simulink model "Model2"  (R2018b)
settings: Solver=ode4  StartTime=0.0  StopTime=tend  FixedStep=dt  RelTol=1e-3
values from neighbouring files (symbols this model uses):
  Bm = 8.6457e-06    [CompareMeasurementModel.m]    (also in ForcedResponse.m; StateSpaceFix.m; SystemEstimateFullN.m; SystemEstimateGammaN.m = 0.0040665)
  Dc = 9.4912e-6    (= 9.4912e-06)    [CompareMeasurementModel.m]    (also in ForcedResponse.m = 8.0176e-06; StateSpaceFix.m = 8.0176e-06; SystemEstimateFullN.m = 0)
  F = 1.3447e-07    [CompareMeasurementModel.m]    (also in ForcedResponse.m; StateSpaceFix.m; SystemEstimateFullN.m; SystemEstimateGammaN.m = 6.3647e-07)
  Freq = 2    [ForcedResponse.m]    (also in StateSpaceFix.m = 1)
  gamma = 1.4811e-09    [CompareMeasurementModel.m]    (also in ForcedResponse.m; StateSpaceFix.m; SystemEstimateFullN.m; SystemEstimateGammaN.m = 8.9133e-10)
  I = 0.012124    [CompareMeasurementModel.m]    (also in ForcedResponse.m = 0.00046323; StateSpaceFix.m = 0.00046323; SystemEstimateFullN.m = 0)
  init = [0 ;0 ;0]    [CompareMeasurementModel.m]    (also in ForcedResponse.m; StateSpaceFix.m; SystemEstimateFullN.m; SystemEstimateGammaN.m = [Pplot(1,1)/(Rg*T/V0) ;0 ;0])
  Jm = 3.0991e-09    [CompareMeasurementModel.m]    (also in ForcedResponse.m; StateSpaceFix.m; SystemEstimateFullN.m; SystemEstimateGammaN.m = 0.00030736)
  L = 0.509    [CompareMeasurementModel.m]    (also in ForcedResponse.m; StateSpaceFix.m; SystemEstimateFullN.m; SystemEstimateGammaN.m)
  N = 73.6905    [CompareMeasurementModel.m]    (also in ForcedResponse.m = 8.8595; StateSpaceFix.m = 8.8595; SystemEstimateFullN.m = 1)
  P = 0.0011648    [CompareMeasurementModel.m]    (also in ForcedResponse.m = 0.00015249; StateSpaceFix.m = 0.00015249; SystemEstimateFullN.m = 1)
  Pend = 1000    [CompareMeasurementModel.m]    (also in ForcedResponse.m = 20000; StateSpaceFix.m = 30000; SystemEstimateFullN.m = 100)
  Period = Tpc*SampleRate*2    (= 20)    [CompareMeasurementModel.m]    (also in ForcedResponse.m = 25; StateSpaceFix.m = 25; SystemEstimateFullN.m; SystemEstimateGammaN.m)
  RatedRatio = 0.0049254    [CompareMeasurementModel.m]    (also in ForcedResponse.m; StateSpaceFix.m; SystemEstimateFullN.m)
  Res = 10    [CompareMeasurementModel.m]    (also in ForcedResponse.m; StateSpaceFix.m; SystemEstimateFullN.m; SystemEstimateGammaN.m)
  Rg = 287.058    [CompareMeasurementModel.m]    (also in ForcedResponse.m; StateSpaceFix.m; SystemEstimateFullN.m; SystemEstimateGammaN.m)
  T = 293.15    [CompareMeasurementModel.m]    (also in ForcedResponse.m; StateSpaceFix.m; SystemEstimateFullN.m; SystemEstimateGammaN.m)
  tau0 = RatedRatio    (= 0.0049254)    [CompareMeasurementModel.m]    (also in ForcedResponse.m; StateSpaceFix.m; SystemEstimateFullN.m; SystemEstimateGammaN.m = 0.53226)
  tstart = Tplot(k-Start+1,1)    [CompareMeasurementModel.m]    (also in ForcedResponse.m = 1; StateSpaceFix.m = 1; SystemEstimateFullN.m; SystemEstimateGammaN.m = 0)
  V0 = 7.658796956e-5    (= 7.658796956e-05)    [CompareMeasurementModel.m]    (also in ForcedResponse.m; StateSpaceFix.m; SystemEstimateFullN.m; SystemEstimateGammaN.m)
  Vboundlower = 0    [ForcedResponse.m]    (also in StateSpaceFix.m)
  Vboundupper = 5    [ForcedResponse.m]    (also in StateSpaceFix.m)
  Vend = V    [CompareMeasurementModel.m]    (also in ForcedResponse.m = 1.5; StateSpaceFix.m = 1.5; SystemEstimateFullN.m; SystemEstimateGammaN.m = 0)
  Vr = 1    [CompareMeasurementModel.m]    (also in ForcedResponse.m; StateSpaceFix.m; SystemEstimateFullN.m; SystemEstimateGammaN.m = 5.48)
  Vs = 1.3    [ForcedResponse.m]    (also in StateSpaceFix.m; SystemEstimateGammaN.m)
  Z = 1.553807*10^(-6)    (= 1.553807e-06)    [CompareMeasurementModel.m]    (also in ForcedResponse.m; StateSpaceFix.m; SystemEstimateFullN.m; SystemEstimateGammaN.m)
libraries: simulink x7
settings Model: Creator=s152155  LastModifiedBy=s152155

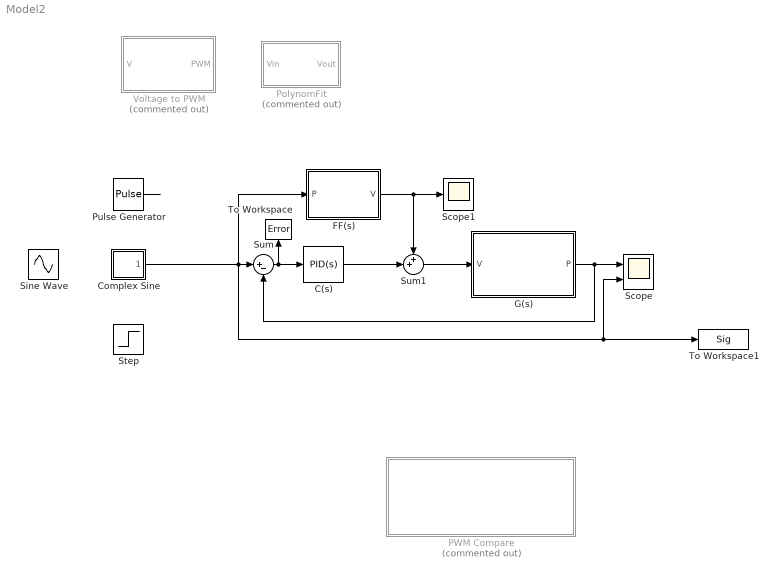
== system Model2 ==
  C(s) : simulink/Continuous/PID Controller  Controller=PID  Form=Parallel  TimeDomain=Continuous-time  SampleTime=-1  IntegratorMethod=Forward Euler  FilterMethod=Forward Euler  ControllerParametersSource=internal  P=P  I=I  D=Dc  UseFilter=on  N=N  TunerSelectOption=Transfer Function Based (PID Tuner App)  InitialConditionSource=internal  InitialConditionForIntegrator=0  InitialConditionForFilter=0  DifferentiatorICPrevScaledInput=0  ExternalReset=none  TrackingMode=off  Kt=1  LimitOutput=off  UpperSaturationLimit=inf  LowerSaturationLimit=-inf  LinearizeAsGain=on  AntiWindupMode=none  Kb=1  POutMin=[]  POutMax=[]  IOutMin=[]  IOutMax=[]  DOutMin=[]  DOutMax=[]  NOutMin=[0]  NOutMax=[0]  SumOutMin=[]  SumOutMax=[]  SaturationOutMin=[]  SaturationOutMax=[]  PParamMin=[]  PParamMax=[]  IParamMin=[]  IParamMax=[]  DParamMin=[]  DParamMax=[]  NParamMin=[]  NParamMax=[]  KbParamMin=[]  KbParamMax=[]  KtParamMin=[]  KtParamMax=[]  KbOutMin=[]  KbOutMax=[]  KtOutMin=[]  KtOutMax=[]  IntegratorOutMin=[]  IntegratorOutMax=[]  FilterOutMin=[]  FilterOutMax=[]  SumI1OutMin=[]  SumI1OutMax=[]  SumI2OutMin=[]  SumI2OutMax=[]  SumI3OutMin=[]  SumI3OutMax=[]  SumI4OutMin=[]  SumI4OutMax=[]  SumDOutMin=[]  SumDOutMax=[]  DifferentiatorOutMin=[]  DifferentiatorOutMax=[]  FilterDiffOutCoefMin=[]  FilterDiffOutCoefMax=[]  ReciprocalOutMin=[]  ReciprocalOutMax=[]  SumDenOutMin=[]  SumDenOutMax=[]  SumNumOutMin=[]  SumNumOutMax=[]  DivideOutMin=[]  DivideOutMax=[]  IntegratorContinuousStateAttributes=''  IntegratorStateMustResolveToSignalObject=off  IntegratorRTWStateStorageClass=Auto  FilterContinuousStateAttributes=''  FilterStateMustResolveToSignalObject=off  FilterRTWStateStorageClass=Auto  ParallelPVariant=InternalParameters  IdealPVariant=Disabled  IVariant=InternalParameters  DVariant=InternalParameters  IntegratorVariant=Continuous  SatVariant=Disabled  AWVariant=Passthrough  PCopyVariant=Disabled  TRVariant=Disabled  FdbkBlocksVariant=Forward  IdealPFdbkVariant=Disabled  SatFdbkVariant=Disabled  DerivativeFilterVariant=ContFilter  NVariant=InternalParameters  NCopyVariant=Disabled  FilterICVariant=InternalICsFilter  IntegratorICVariant=InternalICs  ExternalResetVariant=Disabled  TRSumVariant=Passthrough  SumFdbkVariant=Disabled  SumVariant=Sum_PID
  "Complex Sine " : Subsystem
  FF(s) : Subsystem
  G(s) : Subsystem
  PWM Compare : Subsystem  Commented=on
  "PolynomFit " : Subsystem  Commented=on
  Pulse Generator : DiscretePulseGenerator  PulseType=Time based  Amplitude=Vend  Period=Period  PulseWidth=50  PhaseDelay=tstart
  Scope : Scope  NumInputPorts=2
  Scope1 : Scope
  Sine Wave : Sin  Amplitude=Pend/2  Bias=Pend/2  Frequency=Freq  SampleTime=0
  Step : Step  Time=tstart  After=Pend  SampleTime=0
  Sum : Sum  Inputs=|+-
  Sum1 : Sum  Inputs=++|
  To Workspace : ToWorkspace  VariableName=Error  SaveFormat=Timeseries  SampleTime=-1
  To Workspace1 : ToWorkspace  VariableName=Sig  SaveFormat=Timeseries  SampleTime=-1
  Voltage to PWM : Subsystem  Commented=on
  wires:
  G(s)/1(P) -> Scope/1, Sum/2
  "Complex Sine "/1(Pref) -> To Workspace1/1, Scope/2, FF(s)/1(P), Sum/1
  Sum/1 -> C(s)/1, To Workspace/1
  C(s)/1 -> Sum1/2
  Pulse Generator/1 -> ?
  FF(s)/1(V) -> Sum1/1, Scope1/1
  Sum1/1 -> G(s)/1(V)

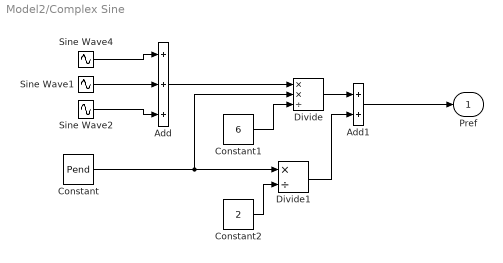
== system Model2/Complex Sine  ==
  Add : Sum  Inputs=3
  Add1 : Sum
  Constant : Constant  Value=Pend
  Constant1 : Constant  Value=6
  Constant2 : Constant  Value=2
  Divide : Product  Inputs=**/
  Divide1 : Product  Inputs=*/
  Sine Wave1 : Sin  Frequency=2*Freq  SampleTime=0
  Sine Wave2 : Sin  Frequency=3*Freq  SampleTime=0
  Sine Wave4 : Sin  Frequency=Freq  SampleTime=0
  Pref : Outport
  wires:
  Divide1/1 -> Add1/2
  Constant/1 -> Divide/2, Divide1/1
  Sine Wave2/1 -> Add/3
  Constant1/1 -> Divide/3
  Sine Wave4/1 -> Add/1
  Sine Wave1/1 -> Add/2
  Divide/1 -> Add1/1
  Constant2/1 -> Divide1/2
  Add/1 -> Divide/1
  Add1/1 -> Pref/1

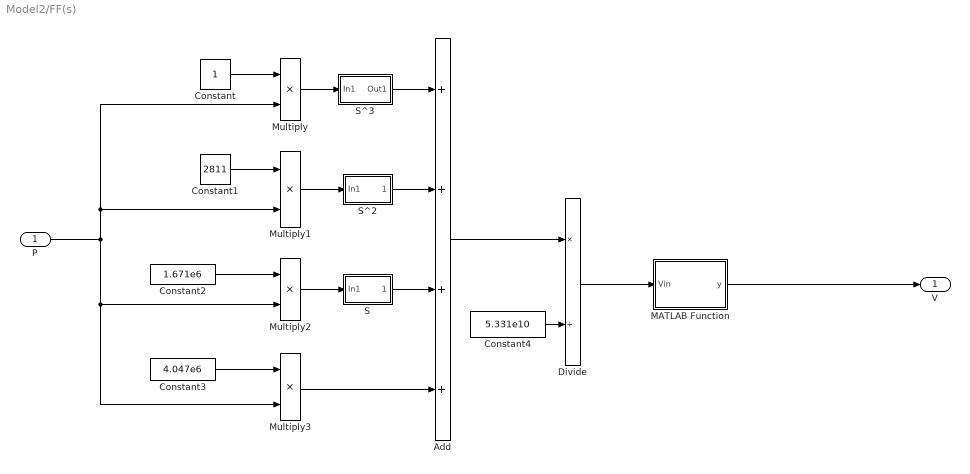
== system Model2/FF(s) ==
  P : Inport
  Add : Sum  Inputs=4
  Constant : Constant
  Constant1 : Constant  Value=2811
  Constant2 : Constant  Value=1.671e6
  Constant3 : Constant  Value=4.047e6
  Constant4 : Constant  Value=5.331e10
  Divide : Product  Inputs=*/
  MATLAB Function : MATLAB Function  TreatAsAtomicUnit=on
  Multiply{,1..3} (4 alike) : Product
  S : Subsystem
  S^2 : Subsystem
  S^3 : Subsystem
  V : Outport
  wires:
  S^3/1(Out1) -> Add/1
  S^2/1(Out1) -> Add/2
  S/1(Out1) -> Add/3
  Constant3/1 -> Multiply3/1
  Constant2/1 -> Multiply2/1
  Constant1/1 -> Multiply1/1
  Constant/1 -> Multiply/1
  Constant4/1 -> Divide/2
  Add/1 -> Divide/1
  P/1 -> Multiply3/2, Multiply2/2, Multiply1/2, Multiply/2
  Multiply/1 -> S^3/1(In1)
  Multiply1/1 -> S^2/1(In1)
  Multiply2/1 -> S/1(In1)
  Multiply3/1 -> Add/4
  Divide/1 -> MATLAB Function/1(Vin)
  MATLAB Function/1(y) -> V/1

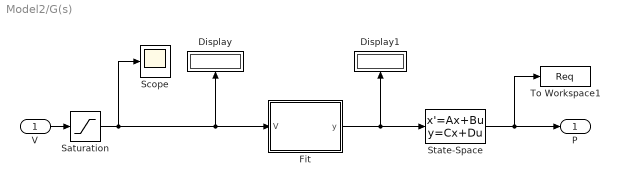
== system Model2/G(s) ==
  V : Inport
  Display : Display
  Display1 : Display
  Fit : MATLAB Function  TreatAsAtomicUnit=on
  Saturation : Saturate  UpperLimit=Vboundupper  LowerLimit=Vboundlower
  Scope : Scope
  State-Space : StateSpace  A=[-gamma*Rg*T/V0 0 Z; 0 -Res/L -Res*RatedRatio/(L); -(F/Jm)*(Rg*T/V0) Res*RatedRatio/(Jm) -Bm/Jm]  B=[0; 1/L; 0]  C=[Rg*T/V0 0 0]  D=0  InitialCondition=init  ContinuousStateAttributes="{'mass',  'current', 'rotationalvelocity'}"
  To Workspace1 : ToWorkspace  VariableName=Req  SaveFormat=Timeseries  SampleTime=-1
  P : Outport
  wires:
  State-Space/1 -> To Workspace1/1, P/1
  V/1 -> Saturation/1
  Saturation/1 -> Scope/1, Display/1, Fit/1(V)
  Fit/1(y) -> Display1/1, State-Space/1

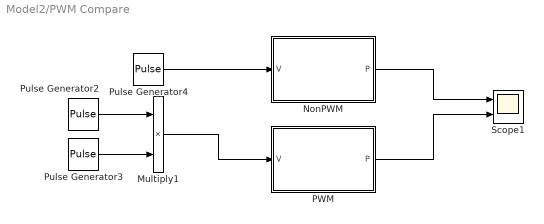
== system Model2/PWM Compare ==
  " NonPWM" : Subsystem
  Multiply1 : Product
  PWM : Subsystem
  Pulse Generator2 : DiscretePulseGenerator  PulseType=Time based  Amplitude=5  Period=25  PulseWidth=50
  Pulse Generator3 : DiscretePulseGenerator  PulseType=Time based  Period=0.01  PulseWidth=60
  Pulse Generator4 : DiscretePulseGenerator  PulseType=Time based  Amplitude=3  Period=Period  PulseWidth=50
  Scope1 : Scope  NumInputPorts=2
  wires:
  Multiply1/1 -> PWM/1(V)
  Pulse Generator3/1 -> Multiply1/2
  Pulse Generator2/1 -> Multiply1/1
  PWM/1(P) -> Scope1/2
  " NonPWM"/1(P) -> Scope1/1
  Pulse Generator4/1 -> " NonPWM"/1(V)

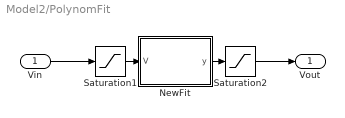
== system Model2/PolynomFit  ==
  Vin : Inport
  "NewFit " : MATLAB Function  TreatAsAtomicUnit=on
  Saturation1 : Saturate  UpperLimit=5  LowerLimit=1.35
  Saturation2 : Saturate  UpperLimit=inf  LowerLimit=0
  Vout : Outport
  wires:
  Saturation1/1 -> "NewFit "/1(V)
  "NewFit "/1(y) -> Saturation2/1
  Vin/1 -> Saturation1/1
  Saturation2/1 -> Vout/1

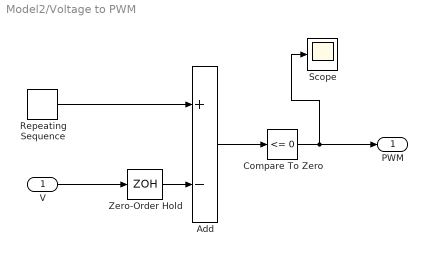
== system Model2/Voltage to PWM ==
  V : Inport
  Add : Sum  Inputs=+-
  Compare To Zero : simulink/Logic and Bit Operations/Compare To Zero  relop=<=  OutDataTypeStr=boolean
  Repeating Sequence : simulink/Sources/Repeating Sequence  rep_seq_t=[0 1]  rep_seq_y=[0 1]
  Scope : Scope
  Zero-Order Hold : ZeroOrderHold  SampleTime=-1
  PWM : Outport
  wires:
  V/1 -> Zero-Order Hold/1
  Zero-Order Hold/1 -> Add/2
  Add/1 -> Compare To Zero/1
  Compare To Zero/1 -> Scope/1, PWM/1
  Repeating Sequence/1 -> Add/1

== system Model2/FF(s)/S ==
  In1 : Inport
  Derivative5 : Derivative
  Out1 : Outport
  wires:
  Derivative5/1 -> Out1/1
  In1/1 -> Derivative5/1

== system Model2/FF(s)/S^2 ==
  In1 : Inport
  Derivative3 : Derivative
  Derivative4 : Derivative
  Out1 : Outport
  wires:
  Derivative4/1 -> Out1/1
  Derivative3/1 -> Derivative4/1
  In1/1 -> Derivative3/1

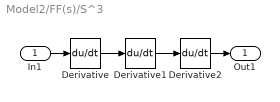
== system Model2/FF(s)/S^3 ==
  In1 : Inport
  Derivative : Derivative
  Derivative1 : Derivative
  Derivative2 : Derivative
  Out1 : Outport
  wires:
  Derivative2/1 -> Out1/1
  Derivative1/1 -> Derivative2/1
  In1/1 -> Derivative/1
  Derivative/1 -> Derivative1/1

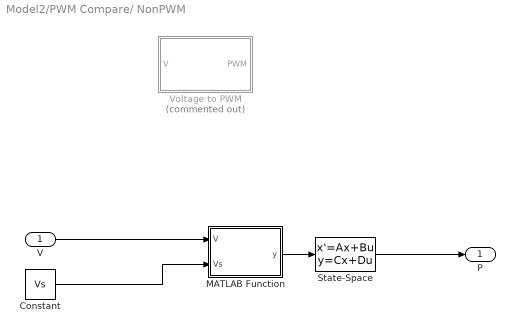
== system Model2/PWM Compare/ NonPWM ==
  V : Inport
  Constant : Constant  Value=Vs
  MATLAB Function : MATLAB Function  TreatAsAtomicUnit=on
  State-Space : StateSpace  A=[-gamma*Rg*T/V0 0 Z; 0 -Res/L -Res*tau0/(L*Vr); -(F/Jm)*(Rg*T/V0) Res*tau0/(Jm*Vr) -Bm/Jm]  B=[0; 1/L; 0]  C=[Rg*T/V0 0 0]  D=0  InitialCondition=init  ContinuousStateAttributes="{'mass',  'current', 'rotationalvelocity'}"
  Voltage to PWM : Subsystem  Commented=on
  P : Outport
  wires:
  State-Space/1 -> P/1
  MATLAB Function/1(y) -> State-Space/1
  V/1 -> MATLAB Function/1(V)
  Constant/1 -> MATLAB Function/2(Vs)

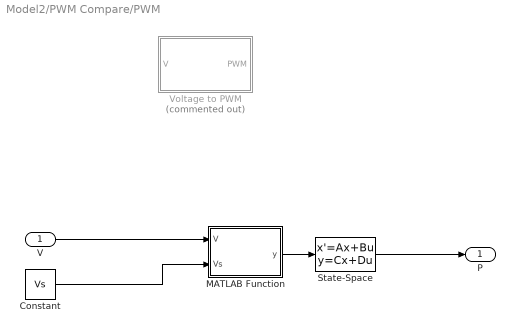
== system Model2/PWM Compare/PWM ==
  V : Inport
  Constant : Constant  Value=Vs
  MATLAB Function : MATLAB Function  TreatAsAtomicUnit=on
  State-Space : StateSpace  A=[-gamma*Rg*T/V0 0 Z; 0 -Res/L -Res*tau0/(L*Vr); -(F/Jm)*(Rg*T/V0) Res*tau0/(Jm*Vr) -Bm/Jm]  B=[0; 1/L; 0]  C=[Rg*T/V0 0 0]  D=0  InitialCondition=init  ContinuousStateAttributes="{'mass',  'current', 'rotationalvelocity'}"
  Voltage to PWM : Subsystem  Commented=on
  P : Outport
  wires:
  State-Space/1 -> P/1
  MATLAB Function/1(y) -> State-Space/1
  V/1 -> MATLAB Function/1(V)
  Constant/1 -> MATLAB Function/2(Vs)

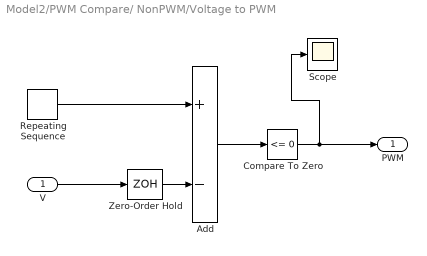
== system Model2/PWM Compare/ NonPWM/Voltage to PWM ==
  V : Inport
  Add : Sum  Inputs=+-
  Compare To Zero : simulink/Logic and Bit Operations/Compare To Zero  relop=<=  OutDataTypeStr=boolean
  Repeating Sequence : simulink/Sources/Repeating Sequence  rep_seq_t=[0 1]  rep_seq_y=[0 1]
  Scope : Scope
  Zero-Order Hold : ZeroOrderHold  SampleTime=-1
  PWM : Outport
  wires:
  V/1 -> Zero-Order Hold/1
  Zero-Order Hold/1 -> Add/2
  Add/1 -> Compare To Zero/1
  Compare To Zero/1 -> Scope/1, PWM/1
  Repeating Sequence/1 -> Add/1

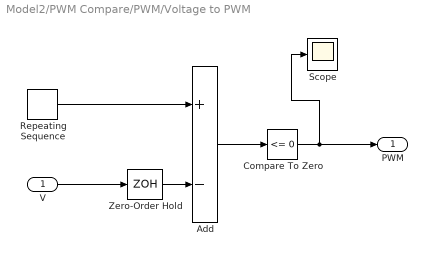
== system Model2/PWM Compare/PWM/Voltage to PWM ==
  V : Inport
  Add : Sum  Inputs=+-
  Compare To Zero : simulink/Logic and Bit Operations/Compare To Zero  relop=<=  OutDataTypeStr=boolean
  Repeating Sequence : simulink/Sources/Repeating Sequence  rep_seq_t=[0 1]  rep_seq_y=[0 1]
  Scope : Scope
  Zero-Order Hold : ZeroOrderHold  SampleTime=-1
  PWM : Outport
  wires:
  V/1 -> Zero-Order Hold/1
  Zero-Order Hold/1 -> Add/2
  Add/1 -> Compare To Zero/1
  Compare To Zero/1 -> Scope/1, PWM/1
  Repeating Sequence/1 -> Add/1

== matlab function Model2/PWM Compare/ NonPWM/MATLAB Function ==
  data: V input; y output; Vs input
function y = Vmin(V, Vs)
if V >= Vs
elseif V<Vs
    V = 0;
elseif V<-Vs
    V = -V;
end
y = V;

== matlab function Model2/G(s)/Fit ==
  data: V input; y output
function y = Vmin(V)
z = 15000;
if V >= 1.1
elseif V<1.1
    V = 0;
elseif V<-1.1
    V = -V;
end

if V >= 1.35
if V<= 2.2
        V = z*(V-1.35)^2;
        if V < 0
            V = 0;
        end
elseif V<= 5
        x = 38000;
        V = x*V - x*2.2 + z*(2.2-1.35)^2;
end
end
V = V *(5/80000);
y = V;

== matlab function Model2/PWM Compare/PWM/MATLAB Function ==
  data: V input; y output; Vs input
function y = Vmin(V, Vs)
if V >= Vs
elseif V<Vs
    V = 0;
elseif V<-Vs
    V = -V;
end
y = V;

== matlab function Model2/PolynomFit /NewFit  ==
  data: V input; y output
function y = Vreal(V)    
    %% Robustness LAR
       p1 =    0.001971;
       p2 =     -0.0458;
       p3 =      0.4358;
       p4 =      -2.163;
       p5 =       5.875;
       p6 =      -8.336;
       p7 =       5.729;
       p8 =      -1.615;
       p9 =      0.1197;


  V = p1*V^8 + p2*V^7 + p3*V^6 + p4*V^5 + p5*V^4 + p6*V^3 + p7*V^2 + p8*V + p9;
y = V;

== matlab function Model2/FF(s)/MATLAB Function ==
  data: Vin input; y output
function y = fcn(Vin)  
    if Vin <= 0
        Vout = 0;
    elseif Vin <= 0.6773
        Vout =  1.032295606*sqrt(Vin)+1.35;
    else
    Vout = (1/2.375)*Vin+ 1.9149;
    end
y = Vout;
